simulink model "MNA5_sim"  (R2014a)
settings: Solver=ode45  StartTime=0.0  StopTime=100  RelTol=1e-3
values from neighbouring files (symbols this model uses):
  MNA5_sys = sys_class    [create_all_sys.m]
settings Model: Creator=UX31  LastModifiedBy=UX31

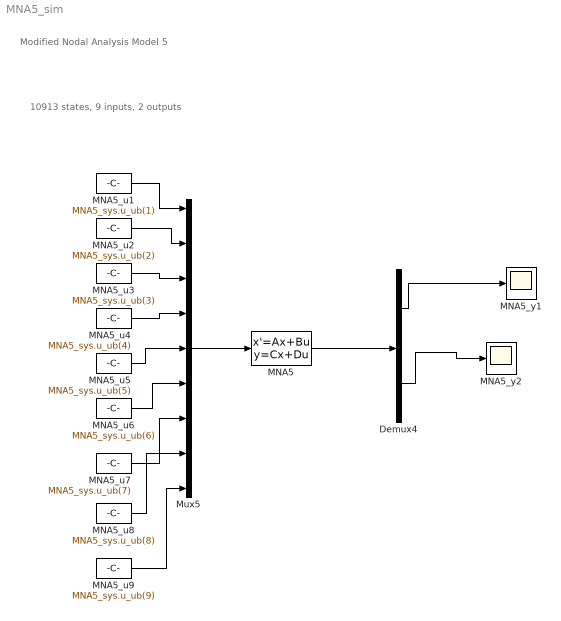
== system MNA5_sim ==
  note: 10913 states, 9 inputs, 2 outputs
  note: Modified Nodal Analysis Model 5
  Demux4 : Demux  Outputs=2
  MNA5 : StateSpace  A=MNA5_sys.sys.a  B=MNA5_sys.sys.b  C=MNA5_sys.sys.c  D=MNA5_sys.sys.d  X0=MNA5_sys.x0_lb
  MNA5_u1 : Constant  Value=MNA5_sys.u_ub(1)
  MNA5_u2 : Constant  Value=MNA5_sys.u_ub(2)
  MNA5_u3 : Constant  Value=MNA5_sys.u_ub(3)
  MNA5_u4 : Constant  Value=MNA5_sys.u_ub(4)
  MNA5_u5 : Constant  Value=MNA5_sys.u_ub(5)
  MNA5_u6 : Constant  Value=MNA5_sys.u_ub(6)
  MNA5_u7 : Constant  Value=MNA5_sys.u_ub(7)
  MNA5_u8 : Constant  Value=MNA5_sys.u_ub(8)
  MNA5_u9 : Constant  Value=MNA5_sys.u_ub(9)
  MNA5_y1 : Scope
      settings: SaveName=ScopeData22
  MNA5_y2 : Scope
      settings: SaveName=ScopeData23
  Mux5 : Mux  Inputs=9
  wires:
  MNA5_u1/1 -> Mux5/1
  MNA5_u2/1 -> Mux5/2
  MNA5_u3/1 -> Mux5/3
  Mux5/1 -> MNA5/1
  MNA5_u4/1 -> Mux5/4
  MNA5_u5/1 -> Mux5/5
  MNA5_u6/1 -> Mux5/6
  MNA5/1 -> Demux4/1
  Demux4/1 -> MNA5_y1/1
  Demux4/2 -> MNA5_y2/1
  MNA5_u7/1 -> Mux5/7
  MNA5_u8/1 -> Mux5/8
  MNA5_u9/1 -> Mux5/9
